simulink model "analogique"  (R2017a)
settings: Solver=FixedStepDiscrete  StartTime=0.0  StopTime=6  RelTol=1e-3  EnableMultiTasking=on
values from neighbouring files (symbols this model uses):
  gainCapteur = 12./max(abs(SortieCapteur(:,2)))    [problematiqueM.m]
libraries: dsparch4 x2, dspsigops x1
settings Model: Creator=dufd2703  LastModifiedBy=Guacamole
settings OptimizationCC: LifeSpan=inf
settings DebuggingCC: SFUnexpectedBacktrackingDiag=warning  SFNoUnconditionalDefaultTransitionDiag=warning  SFExecutionAtInitializationDiag=none
settings GRTTargetCC: TargetLangStandard=C89/C90 (ANSI)  GeneratePreprocessorConditionals=Disable all
settings ConfigComp: CovMetricSettings=dw  CovHtmlReporting=on  CovSaveCumulativeToWorkspaceVar=on  CovSaveSingleToWorkspaceVar=on  CovExternalEMLEnable=off

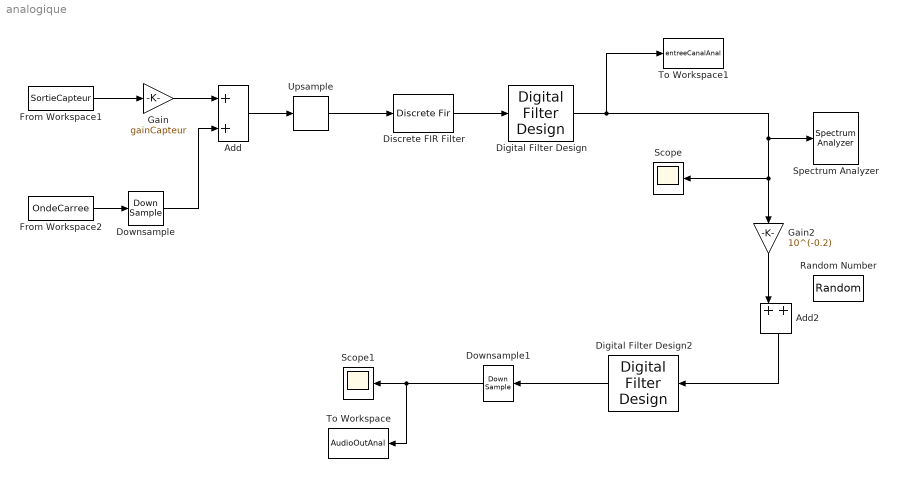
== system analogique ==
  Add : Sum
  Add2 : Sum
  Digital Filter Design : dsparch4/Digital Filter Design  mwdsp_browser_bugfix_var=off
  Digital Filter Design2 : dsparch4/Digital Filter Design  mwdsp_browser_bugfix_var=off
  Discrete FIR Filter : DiscreteFir  Coefficients=ones(1,10)
  Downsample : DownSample  N=3  RateOptions=Allow multirate processing
  Downsample1 : DownSample  N=10  RateOptions=Allow multirate processing
  From Workspace1 : FromWorkspace  VariableName=SortieCapteur  SampleTime=1/16000  Interpolate=off  OutputAfterFinalValue=Setting to zero
  From Workspace2 : FromWorkspace  VariableName=OndeCarree  SampleTime=1/48000  Interpolate=off  OutputAfterFinalValue=Setting to zero
  Gain : Gain  Gain=gainCapteur
  Gain2 : Gain  Gain=10^(-0.2)
  Random Number : RandomNumber  Variance=160000*0.000002  SampleTime=1/160000
  Scope : Scope
  Scope1 : Scope
  Spectrum Analyzer : SpectrumAnalyzer
  To Workspace : ToWorkspace  VariableName=AudioOutAnal  SampleTime=-1
      settings: Save2DSignal=2-D array (concatenate along first dimension)
  To Workspace1 : ToWorkspace  VariableName=entreeCanalAnal  SampleTime=-1
      settings: Save2DSignal=2-D array (concatenate along first dimension)
  Upsample : dspsigops/Upsample  N=10  phase=0  RateOptions=Allow multirate processing  ic=0  mode=Unused parameter value
  wires:
  From Workspace1/1 -> Gain/1
  Gain/1 -> Add/1
  Add/1 -> Upsample/1
  Downsample/1 -> Add/2
  From Workspace2/1 -> Downsample/1
  Discrete FIR Filter/1 -> Digital Filter Design/1
  Upsample/1 -> Discrete FIR Filter/1
  Digital Filter Design/1 -> To Workspace1/1, Scope/1, Gain2/1, Spectrum Analyzer/1
  Digital Filter Design2/1 -> Downsample1/1
  Add2/1 -> Digital Filter Design2/1
  Downsample1/1 -> To Workspace/1, Scope1/1
  Gain2/1 -> Add2/1
